simulink model "cruise_control_001"  (R2019b)
settings: Solver=VariableStepAuto  StartTime=0.0  StopTime=120  RelTol=1e-3
undefined symbols (not defined in the file): b, m
settings Model: Creator=Yinglongli  LastModifiedBy=Yinglongli

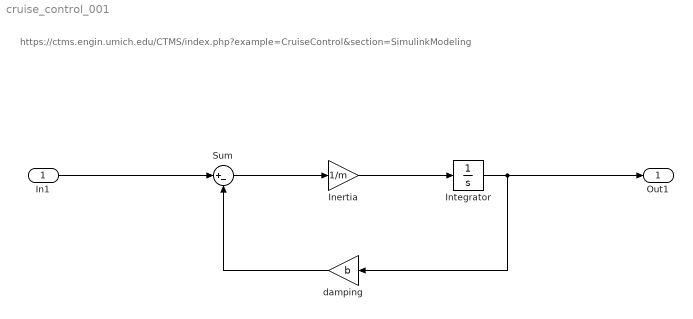
== system cruise_control_001 ==
  note: https://ctms.engin.umich.edu/CTMS/index.php?example=CruiseControl&section=SimulinkModeling
  In1 : Inport
  Inertia : Gain  Gain=1/m
  Integrator : Integrator
  Sum : Sum  Inputs=|+-
  damping : Gain  Gain=b
  Out1 : Outport
  wires:
  Inertia/1 -> Integrator/1
  Sum/1 -> Inertia/1
  Integrator/1 -> Out1/1, damping/1
  damping/1 -> Sum/2
  In1/1 -> Sum/1
